simulink model "custom_springs_ALL"  (R2026a)
settings: Solver=ode23t  StopTime=15  AbsTol=1e-3  EnableMultiTasking=on
InitFcn:
  | warning off Simulink:SL_MatchingFromNotFound
  | m=1;
  | b=1;
  | k=1;
libraries: fl_lib x58, nesl_utility x10
Description:
  | Copyright 2014-2026 The MathWorks, Inc.
settings Model: Creator=tegel  LastModifiedBy=smiller
settings DataIOCC: SignalLoggingSaveFormat=ModelDataLogs
settings OptimizationCC: InitFltsAndDblsToZero=on
settings DebuggingCC: SaveWithParameterizedLinksMsg=none  UnderspecifiedInitializationDetection=Classic
settings HardwareCC: ProdHWDeviceType=32-bit Generic
settings GRTTargetCC: TargetFcnLib=ansi_tfl_tmw.mat  CombineOutputUpdateFcns=off  GRTInterface=on
settings SimscapeCC: SimscapeNormalizeSystem=off  SimscapeNominalValues="[{\"value\":\"1\",\"unit\":\"A\"},{\"value\":\"1\",\"unit\":\"bar\"},{\"value\":\"1\",\"unit\":\"cm^2\"},{\"value\":\"1\",\"unit\":\"cm^3/s\"},{\"value\":\"1\",\"unit\":\"kJ/kg\"},{\"value\":\"1\",\"unit\":\"kW\"},{\"value\":\"1\",\"unit\":\"l\"},{\"value\":\"1\",\"unit\":\"N\"},{\"value\":\"1\",\"unit\":\"N*m\"},{\"value\":\"1\",\"unit\":\"V\"}]"  SimscapeLogType=none  SimscapeLogDataHistory=5000.0

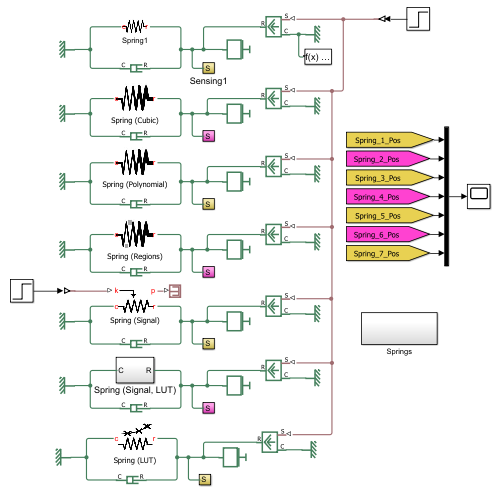
[thumbnail: Simulink's stored preview of the top-level diagram]
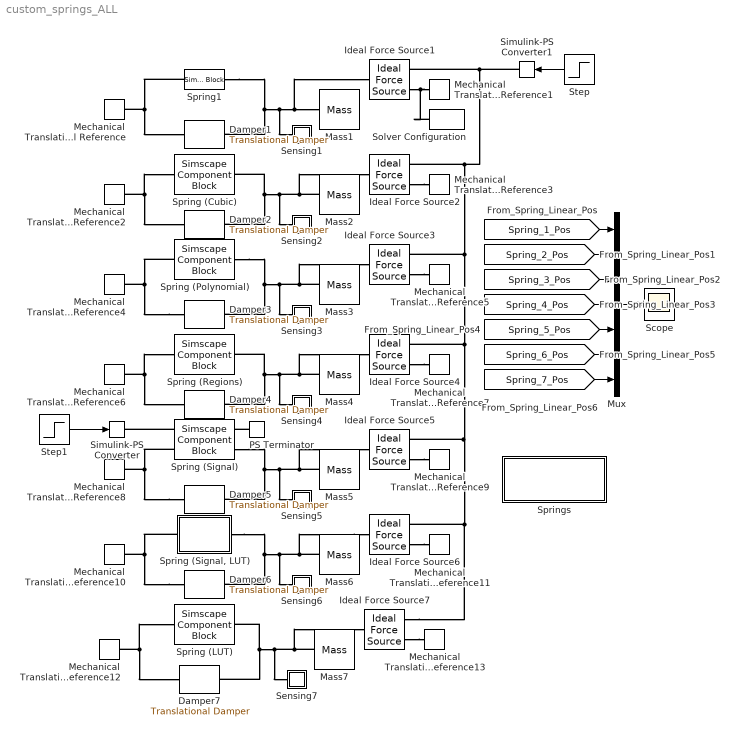
== system custom_springs_ALL ==
  Damper{1..7} (7 alike) : fl_lib/Mechanical/Translational Elements/Translational Damper  D=b N/(m/s)  v_specify=off  v_priority=High  v=0 m/s  v_nominal_specify=off  v_nominal_value=1  v_nominal_unit=m/s  f_specify=off  f_priority=High  f=0 N  f_nominal_specify=off  f_nominal_value=1  f_nominal_unit=N
  Ideal Force Source{1..7} (7 alike) : fl_lib/Mechanical/Mechanical Sources/Ideal Force Source
  Mass{1..7} (7 alike) : fl_lib/Mechanical/Translational Elements/Mass  mass=m kg  num_ports=foundation.enum.numPorts2.one  v_specify=on  v_priority=High  v=0 m/s  v_nominal_specify=off  v_nominal_value=1  v_nominal_unit=m/s  f_specify=off  f_priority=High  f=0 N  f_nominal_specify=off  f_nominal_value=1  f_nominal_unit=N
  Mechanical Translational Reference{,1..13} (14 alike) : fl_lib/Mechanical/Translational Elements/Mechanical Translational Reference
  Mux : Mux  Inputs=7
  PS Terminator : fl_lib/Physical Signals/Sinks/PS Terminator
  Scope : Scope
      settings: TimeSpan=15  ActiveDisplayYMinimum=0  ActiveDisplayYMaximum=2.5  DataLoggingVariableName=Simscape_Language_Spring_DATA
  Sensing1 : Subsystem
  Sensing2 : Subsystem
  Sensing3 : Subsystem
  Sensing4 : Subsystem
  Sensing5 : Subsystem
  Sensing6 : Subsystem
  Sensing7 : Subsystem
  Simulink-PS Converter : nesl_utility/Simulink-PS Converter  PhysicalDomain=network_engine_domain  SubClassName=ps_input  LeftPortType=input  RightPortType=output  PseudoPeriodic=off  Frequencies=[]  NoiseDistribution=none  NoiseParameters=[]  Unit=1  AffineConversion=off  FilteringAndDerivatives=provide  SimscapeFilterOrder=1  InputFilterTimeConstant=.001  UdotUserProvided=0
  Simulink-PS Converter1 : nesl_utility/Simulink-PS Converter  PhysicalDomain=network_engine_domain  SubClassName=ps_input  LeftPortType=input  RightPortType=output  PseudoPeriodic=off  Frequencies=[]  NoiseDistribution=none  NoiseParameters=[]  Unit=1  AffineConversion=off  FilteringAndDerivatives=provide  SimscapeFilterOrder=1  InputFilterTimeConstant=.001  UdotUserProvided=0
  Solver Configuration : nesl_utility/Solver Configuration  PhysicalDomain=network_engine_domain  SubClassName=solver  LeftPortType=input  RightPortType=generic  Tones=[]  Harmonics=[]  SimulateNoise=off  Profile=off  UseLocalSampling=off  EnableSwitchedLinearOptims=on  FrequencyDomain=off  UseCCode=off  RelTol=0.001  AbsTol=1e-06  MinStep=1e-09  ToWorkspace=off  RevertToSquareIcSolve=off  NumHomotopyIterations=100  PhasorMode=off  PhasorModeNumHarmonics=1  ConsistencySolver=NEWTON_FTOL  CanonicalOrdering=UNORDERED  OptimizeIntermediates=UNOPTIMIZED  IndexReductionMethod=DerivativeReplacement  DoDC=off  ResidualTolerance=1e-9  ConsistencyTolSource=GLOBAL  ConsistencyAbsTol=0.001  ConsistencyRelTol=0.001  ConsistencyTolFactor=0.001  UseLocalSolver=off  LocalSolverChoice=NE_BACKWARD_EULER_ADVANCER  ResolveIndetEquations=on  FunctionEvalNumThread=1  LocalSolverSampleTime=.001  DoFixedCost=off  MaxNonlinIter=3  MaxModeIter=2  ComputeImpulses=off  ImpulseIterations=2  LinearAlgebra=Sparse  LinearAlgebraNumThread=0  EquationFormulation=NE_TIME_EF  DelaysMemoryBudget=1024  AutomaticFiltering=on  FilteringTimeConstant=0.001  PartitionStorageMethod=AS_NEEDED  PartitionMemoryBudget=1024  PartitionMethod=FAST  MultibodyUseLocalSolver=off  MultibodyLocalSolverChoice=ODE1  MultibodyLocalSolverSampleTime=0.001
  Spring (Cubic) : SimscapeComponentBlock  SourceFile=CustomSprings.SpringCubic  ComponentPath=CustomSprings.SpringCubic  ComponentVariants=CustomSprings.SpringCubic  ComponentVariantNames=SpringCubic  ClassName=SpringCubic  SchemaVersion=1  k=1 N/m^3  v_specify=off  v_priority=None  v=0 m/s  v_nominal_specify=off  v_nominal_value=1  v_nominal_unit=m/s  f_specify=off  f_priority=None  f=0 N  f_nominal_specify=off  f_nominal_value=1  f_nominal_unit=N  x_specify=off  x_priority=None  x=0 m  x_nominal_specify=off  x_nominal_value=1  x_nominal_unit=m
      settings: CopyFcn=simscape.sscblock.internal.componentBlockCallback(gcbh,'COPY')  PreCopyFcn=simscape.sscblock.internal.componentBlockCallback(gcbh,'PRECOPY')  PreDeleteFcn=simscape.sscblock.internal.componentBlockCallback(gcbh,'PREDELETE')
      mask Type: Spring (Cubic)
  Spring (LUT) : SimscapeComponentBlock  SourceFile=CustomSprings.SpringLUT  ComponentPath=CustomSprings.SpringLUT  ComponentVariants=CustomSprings.SpringLUT  ComponentVariantNames=SpringLUT  ClassName=SpringLUT  SchemaVersion=1  xd=[-4.0, -3.0, -2.0, -1.0, 0.0, 1.0, 2.0, 3.0, 4.0] m  kd=[1000000.0, 8.0, 4.0, 2.0, 0.0, 2.0, 4.0, 8.0, 1000000.0] N/m  v_specify=off  v_priority=None  v=0 m/s  v_nominal_specify=off  v_nominal_value=1  v_nominal_unit=m/s  f_specify=off  f_priority=None  f=0 N  f_nominal_specify=off  f_nominal_value=1  f_nominal_unit=N  x_specify=off  x_priority=None  x=0 m  x_nominal_specify=off  x_nominal_value=1  x_nominal_unit=m  k_specify=off  k_priority=None  k=0 N/m  k_nominal_specify=off  k_nominal_value=1  k_nominal_unit=N/m
      settings: CopyFcn=simscape.sscblock.internal.componentBlockCallback(gcbh,'COPY')  PreCopyFcn=simscape.sscblock.internal.componentBlockCallback(gcbh,'PRECOPY')  PreDeleteFcn=simscape.sscblock.internal.componentBlockCallback(gcbh,'PREDELETE')
      mask Type: Spring (Lookup Table)
  Spring (Polynomial) : SimscapeComponentBlock  SourceFile=CustomSprings.SpringPolynomial  ComponentPath=CustomSprings.SpringPolynomial  ComponentVariants=CustomSprings.SpringPolynomial  ComponentVariantNames=SpringPolynomial  ClassName=SpringPolynomial  SchemaVersion=1  k=1 N/m  k1=1 N/m^3  v_specify=off  v_priority=None  v=0 m/s  v_nominal_specify=off  v_nominal_value=1  v_nominal_unit=m/s  f_specify=off  f_priority=None  f=0 N  f_nominal_specify=off  f_nominal_value=1  f_nominal_unit=N  x_specify=off  x_priority=None  x=0 m  x_nominal_specify=off  x_nominal_value=1  x_nominal_unit=m
      settings: CopyFcn=simscape.sscblock.internal.componentBlockCallback(gcbh,'COPY')  PreCopyFcn=simscape.sscblock.internal.componentBlockCallback(gcbh,'PRECOPY')  PreDeleteFcn=simscape.sscblock.internal.componentBlockCallback(gcbh,'PREDELETE')
      mask Type: Spring (Polynomial)
  Spring (Regions) : SimscapeComponentBlock  SourceFile=CustomSprings.SpringRegions  ComponentPath=CustomSprings.SpringRegions  ComponentVariants=CustomSprings.SpringRegions  ComponentVariantNames=SpringRegions  ClassName=SpringRegions  SchemaVersion=1  k=1 N/m  k1=1 N/m^3  xc=0.2 m  v_specify=off  v_priority=None  v=0 m/s  v_nominal_specify=off  v_nominal_value=1  v_nominal_unit=m/s  f_specify=off  f_priority=None  f=0 N  f_nominal_specify=off  f_nominal_value=1  f_nominal_unit=N  x_specify=off  x_priority=None  x=0 m  x_nominal_specify=off  x_nominal_value=1  x_nominal_unit=m
      settings: CopyFcn=simscape.sscblock.internal.componentBlockCallback(gcbh,'COPY')  PreCopyFcn=simscape.sscblock.internal.componentBlockCallback(gcbh,'PRECOPY')  PreDeleteFcn=simscape.sscblock.internal.componentBlockCallback(gcbh,'PREDELETE')
      mask Type: Spring (Regions)
  Spring (Signal) : SimscapeComponentBlock  SourceFile=CustomSprings.SpringSignal  ComponentPath=CustomSprings.SpringSignal  ComponentVariants=CustomSprings.SpringSignal  ComponentVariantNames=SpringSignal  ClassName=SpringSignal  SchemaVersion=1  v_specify=off  v_priority=None  v=0 m/s  v_nominal_specify=off  v_nominal_value=1  v_nominal_unit=m/s  f_specify=off  f_priority=None  f=0 N  f_nominal_specify=off  f_nominal_value=1  f_nominal_unit=N  x_specify=off  x_priority=None  x=0 m  x_nominal_specify=off  x_nominal_value=1  x_nominal_unit=m
      settings: CopyFcn=simscape.sscblock.internal.componentBlockCallback(gcbh,'COPY')  PreCopyFcn=simscape.sscblock.internal.componentBlockCallback(gcbh,'PRECOPY')  PreDeleteFcn=simscape.sscblock.internal.componentBlockCallback(gcbh,'PREDELETE')
      mask Type: Spring (Signal)
  "Spring (Signal, LUT)" : Subsystem
  Spring1 : SimscapeComponentBlock  SourceFile=CustomSprings.SpringLinear  ComponentPath=CustomSprings.SpringLinear  ComponentVariants=CustomSprings.SpringLinear  ComponentVariantNames=SpringLinear  ClassName=SpringLinear  SchemaVersion=1  k=1 N/m  v_specify=off  v_priority=None  v=0 m/s  v_nominal_specify=off  v_nominal_value=1  v_nominal_unit=m/s  f_specify=off  f_priority=None  f=0 N  f_nominal_specify=off  f_nominal_value=1  f_nominal_unit=N  x_specify=off  x_priority=None  x=0 m  x_nominal_specify=off  x_nominal_value=1  x_nominal_unit=m
      settings: CopyFcn=simscape.sscblock.internal.componentBlockCallback(gcbh,'COPY')  PreCopyFcn=simscape.sscblock.internal.componentBlockCallback(gcbh,'PRECOPY')  PreDeleteFcn=simscape.sscblock.internal.componentBlockCallback(gcbh,'PREDELETE')
      mask Type: Spring
  Springs : Subsystem
  Step : Step  FinalValue=2  SampleTime=0
  Step1 : Step  Time=10  InitialValue=1  FinalValue=2  SampleTime=0
  wires:
  Mux/1 -> Scope/1
  [Spring_1_Pos] -> Mux/1
  [Spring_2_Pos] -> Mux/2
  Step/1 -> Simulink-PS Converter1/1
  Step1/1 -> Simulink-PS Converter/1
  [Spring_3_Pos] -> Mux/3
  [Spring_4_Pos] -> Mux/4
  [Spring_5_Pos] -> Mux/5
  [Spring_6_Pos] -> Mux/6
  [Spring_7_Pos] -> Mux/7
  connections:
  Ideal Force Source4/RConn1 -- Ideal Force Source3/RConn1 -- Ideal Force Source1/RConn1 -- Simulink-PS Converter1/RConn1 -- Ideal Force Source2/RConn1 -- Ideal Force Source5/RConn1 -- Ideal Force Source6/RConn1 -- Ideal Force Source7/RConn1
  Ideal Force Source1/RConn2 -- Solver Configuration/RConn1 -- Mechanical Translational Reference1/LConn1
  Mechanical Translational Reference/LConn1 -- Spring1/LConn1 -- Damper1/RConn1
  Damper1/LConn1 -- Spring1/RConn1 -- Sensing1/LConn1 -- Mass1/LConn1 -- Ideal Force Source1/LConn1
  Mechanical Translational Reference2/LConn1 -- Spring (Cubic)/LConn1 -- Damper2/RConn1
  Damper2/LConn1 -- Spring (Cubic)/RConn1 -- Sensing2/LConn1 -- Mass2/LConn1 -- Ideal Force Source2/LConn1
  Ideal Force Source2/RConn2 -- Mechanical Translational Reference3/LConn1
  Damper3/RConn1 -- Spring (Polynomial)/LConn1 -- Mechanical Translational Reference4/LConn1
  Spring (Polynomial)/RConn1 -- Damper3/LConn1 -- Ideal Force Source3/LConn1 -- Mass3/LConn1 -- Sensing3/LConn1
  Ideal Force Source3/RConn2 -- Mechanical Translational Reference5/LConn1
  Mechanical Translational Reference6/LConn1 -- Spring (Regions)/LConn1 -- Damper4/RConn1
  Damper4/LConn1 -- Spring (Regions)/RConn1 -- Sensing4/LConn1 -- Mass4/LConn1 -- Ideal Force Source4/LConn1
  Ideal Force Source4/RConn2 -- Mechanical Translational Reference7/LConn1
  Damper5/RConn1 -- Spring (Signal)/LConn2 -- Mechanical Translational Reference8/LConn1
  Spring (Signal)/RConn2 -- Damper5/LConn1 -- Ideal Force Source5/LConn1 -- Mass5/LConn1 -- Sensing5/LConn1
  Ideal Force Source5/RConn2 -- Mechanical Translational Reference9/LConn1
  Damper6/RConn1 -- "Spring (Signal, LUT)"/LConn1 -- Mechanical Translational Reference10/LConn1
  Ideal Force Source6/LConn1 -- "Spring (Signal, LUT)"/RConn1 -- Damper6/LConn1 -- Sensing6/LConn1 -- Mass6/LConn1
  Ideal Force Source6/RConn2 -- Mechanical Translational Reference11/LConn1
  Spring (Signal)/LConn1 -- Simulink-PS Converter/RConn1
  Mechanical Translational Reference12/LConn1 -- Spring (LUT)/LConn1 -- Damper7/RConn1
  Damper7/LConn1 -- Spring (LUT)/RConn1 -- Sensing7/LConn1 -- Mass7/LConn1 -- Ideal Force Source7/LConn1
  Ideal Force Source7/RConn2 -- Mechanical Translational Reference13/LConn1
  PS Terminator/LConn1 -- Spring (Signal)/RConn1

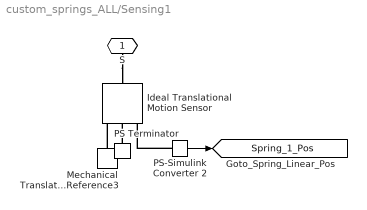
== system custom_springs_ALL/Sensing1 ==
  Ideal Translational Motion Sensor : fl_lib/Mechanical/Mechanical Sensors/Ideal Translational Motion Sensor  reference=foundation.enum.MeasurementReference.difference  acceleration_port=false  velocity_port=true  position_port=true  offset=0 m
  Mechanical Translational Reference3 : fl_lib/Mechanical/Translational Elements/Mechanical Translational Reference
  PS Terminator : fl_lib/Physical Signals/Sinks/PS Terminator
  PS-Simulink Converter 2 : nesl_utility/PS-Simulink Converter  PhysicalDomain=network_engine_domain  SubClassName=ps_output  LeftPortType=input  RightPortType=output  PseudoPeriodic=off  Frequencies=[]  VectorFormat=1-D array  Unit=1  AffineConversion=off
  S : PMIOPort  Side=Left
  tag scope: Spring_1_Pos=global
  wires:
  PS-Simulink Converter 2/1 -> [Spring_1_Pos]
  connections:
  S/RConn1 -- Ideal Translational Motion Sensor/LConn1
  Mechanical Translational Reference3/LConn1 -- Ideal Translational Motion Sensor/RConn1
  PS-Simulink Converter 2/LConn1 -- Ideal Translational Motion Sensor/RConn3
  PS Terminator/LConn1 -- Ideal Translational Motion Sensor/RConn2

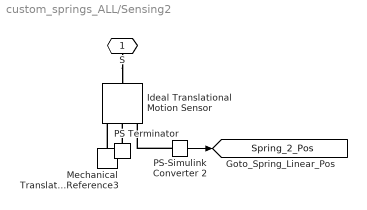
== system custom_springs_ALL/Sensing2 ==
  Ideal Translational Motion Sensor : fl_lib/Mechanical/Mechanical Sensors/Ideal Translational Motion Sensor  reference=foundation.enum.MeasurementReference.difference  acceleration_port=false  velocity_port=true  position_port=true  offset=0 m
  Mechanical Translational Reference3 : fl_lib/Mechanical/Translational Elements/Mechanical Translational Reference
  PS Terminator : fl_lib/Physical Signals/Sinks/PS Terminator
  PS-Simulink Converter 2 : nesl_utility/PS-Simulink Converter  PhysicalDomain=network_engine_domain  SubClassName=ps_output  LeftPortType=input  RightPortType=output  PseudoPeriodic=off  Frequencies=[]  VectorFormat=1-D array  Unit=1  AffineConversion=off
  S : PMIOPort  Side=Left
  tag scope: Spring_2_Pos=global
  wires:
  PS-Simulink Converter 2/1 -> [Spring_2_Pos]
  connections:
  PS-Simulink Converter 2/LConn1 -- Ideal Translational Motion Sensor/RConn3
  Mechanical Translational Reference3/LConn1 -- Ideal Translational Motion Sensor/RConn1
  S/RConn1 -- Ideal Translational Motion Sensor/LConn1
  PS Terminator/LConn1 -- Ideal Translational Motion Sensor/RConn2

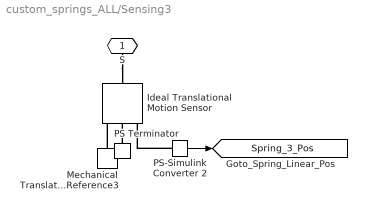
== system custom_springs_ALL/Sensing3 ==
  Ideal Translational Motion Sensor : fl_lib/Mechanical/Mechanical Sensors/Ideal Translational Motion Sensor  reference=foundation.enum.MeasurementReference.difference  acceleration_port=false  velocity_port=true  position_port=true  offset=0 m
  Mechanical Translational Reference3 : fl_lib/Mechanical/Translational Elements/Mechanical Translational Reference
  PS Terminator : fl_lib/Physical Signals/Sinks/PS Terminator
  PS-Simulink Converter 2 : nesl_utility/PS-Simulink Converter  PhysicalDomain=network_engine_domain  SubClassName=ps_output  LeftPortType=input  RightPortType=output  PseudoPeriodic=off  Frequencies=[]  VectorFormat=1-D array  Unit=1  AffineConversion=off
  S : PMIOPort  Side=Left
  tag scope: Spring_3_Pos=global
  wires:
  PS-Simulink Converter 2/1 -> [Spring_3_Pos]
  connections:
  S/RConn1 -- Ideal Translational Motion Sensor/LConn1
  Mechanical Translational Reference3/LConn1 -- Ideal Translational Motion Sensor/RConn1
  PS-Simulink Converter 2/LConn1 -- Ideal Translational Motion Sensor/RConn3
  PS Terminator/LConn1 -- Ideal Translational Motion Sensor/RConn2

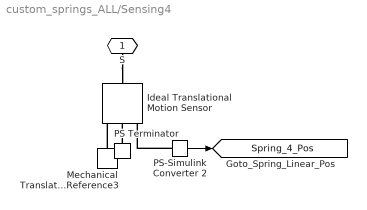
== system custom_springs_ALL/Sensing4 ==
  Ideal Translational Motion Sensor : fl_lib/Mechanical/Mechanical Sensors/Ideal Translational Motion Sensor  reference=foundation.enum.MeasurementReference.difference  acceleration_port=false  velocity_port=true  position_port=true  offset=0 m
  Mechanical Translational Reference3 : fl_lib/Mechanical/Translational Elements/Mechanical Translational Reference
  PS Terminator : fl_lib/Physical Signals/Sinks/PS Terminator
  PS-Simulink Converter 2 : nesl_utility/PS-Simulink Converter  PhysicalDomain=network_engine_domain  SubClassName=ps_output  LeftPortType=input  RightPortType=output  PseudoPeriodic=off  Frequencies=[]  VectorFormat=1-D array  Unit=1  AffineConversion=off
  S : PMIOPort  Side=Left
  tag scope: Spring_4_Pos=global
  wires:
  PS-Simulink Converter 2/1 -> [Spring_4_Pos]
  connections:
  PS-Simulink Converter 2/LConn1 -- Ideal Translational Motion Sensor/RConn3
  Mechanical Translational Reference3/LConn1 -- Ideal Translational Motion Sensor/RConn1
  S/RConn1 -- Ideal Translational Motion Sensor/LConn1
  PS Terminator/LConn1 -- Ideal Translational Motion Sensor/RConn2

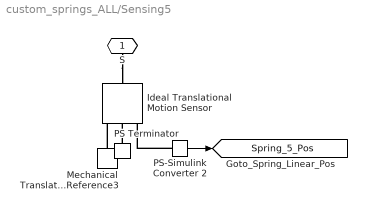
== system custom_springs_ALL/Sensing5 ==
  Ideal Translational Motion Sensor : fl_lib/Mechanical/Mechanical Sensors/Ideal Translational Motion Sensor  reference=foundation.enum.MeasurementReference.difference  acceleration_port=false  velocity_port=true  position_port=true  offset=0 m
  Mechanical Translational Reference3 : fl_lib/Mechanical/Translational Elements/Mechanical Translational Reference
  PS Terminator : fl_lib/Physical Signals/Sinks/PS Terminator
  PS-Simulink Converter 2 : nesl_utility/PS-Simulink Converter  PhysicalDomain=network_engine_domain  SubClassName=ps_output  LeftPortType=input  RightPortType=output  PseudoPeriodic=off  Frequencies=[]  VectorFormat=1-D array  Unit=1  AffineConversion=off
  S : PMIOPort  Side=Left
  tag scope: Spring_5_Pos=global
  wires:
  PS-Simulink Converter 2/1 -> [Spring_5_Pos]
  connections:
  S/RConn1 -- Ideal Translational Motion Sensor/LConn1
  Mechanical Translational Reference3/LConn1 -- Ideal Translational Motion Sensor/RConn1
  PS-Simulink Converter 2/LConn1 -- Ideal Translational Motion Sensor/RConn3
  PS Terminator/LConn1 -- Ideal Translational Motion Sensor/RConn2

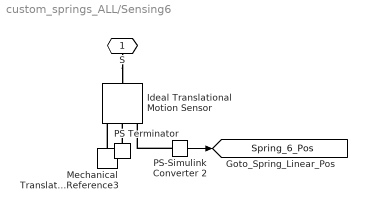
== system custom_springs_ALL/Sensing6 ==
  Ideal Translational Motion Sensor : fl_lib/Mechanical/Mechanical Sensors/Ideal Translational Motion Sensor  reference=foundation.enum.MeasurementReference.difference  acceleration_port=false  velocity_port=true  position_port=true  offset=0 m
  Mechanical Translational Reference3 : fl_lib/Mechanical/Translational Elements/Mechanical Translational Reference
  PS Terminator : fl_lib/Physical Signals/Sinks/PS Terminator
  PS-Simulink Converter 2 : nesl_utility/PS-Simulink Converter  PhysicalDomain=network_engine_domain  SubClassName=ps_output  LeftPortType=input  RightPortType=output  PseudoPeriodic=off  Frequencies=[]  VectorFormat=1-D array  Unit=1  AffineConversion=off
  S : PMIOPort  Side=Left
  tag scope: Spring_6_Pos=global
  wires:
  PS-Simulink Converter 2/1 -> [Spring_6_Pos]
  connections:
  PS-Simulink Converter 2/LConn1 -- Ideal Translational Motion Sensor/RConn3
  Mechanical Translational Reference3/LConn1 -- Ideal Translational Motion Sensor/RConn1
  S/RConn1 -- Ideal Translational Motion Sensor/LConn1
  PS Terminator/LConn1 -- Ideal Translational Motion Sensor/RConn2

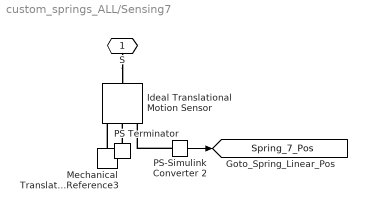
== system custom_springs_ALL/Sensing7 ==
  Ideal Translational Motion Sensor : fl_lib/Mechanical/Mechanical Sensors/Ideal Translational Motion Sensor  reference=foundation.enum.MeasurementReference.difference  acceleration_port=false  velocity_port=true  position_port=true  offset=0 m
  Mechanical Translational Reference3 : fl_lib/Mechanical/Translational Elements/Mechanical Translational Reference
  PS Terminator : fl_lib/Physical Signals/Sinks/PS Terminator
  PS-Simulink Converter 2 : nesl_utility/PS-Simulink Converter  PhysicalDomain=network_engine_domain  SubClassName=ps_output  LeftPortType=input  RightPortType=output  PseudoPeriodic=off  Frequencies=[]  VectorFormat=1-D array  Unit=1  AffineConversion=off
  S : PMIOPort  Side=Left
  tag scope: Spring_7_Pos=global
  wires:
  PS-Simulink Converter 2/1 -> [Spring_7_Pos]
  connections:
  S/RConn1 -- Ideal Translational Motion Sensor/LConn1
  Mechanical Translational Reference3/LConn1 -- Ideal Translational Motion Sensor/RConn1
  PS-Simulink Converter 2/LConn1 -- Ideal Translational Motion Sensor/RConn3
  PS Terminator/LConn1 -- Ideal Translational Motion Sensor/RConn2

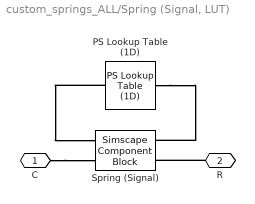
== system custom_springs_ALL/Spring (Signal, LUT) ==
  PS Lookup Table (1D) : fl_lib/Physical Signals/Lookup Tables/PS Lookup Table (1D)  x=[-4 -3 -2 -1 0 1 2 3 4] m  f=[1e6 8 4 2 0 2 4 8 1e6] N/m  interp_method=simscape.enum.interpolation.linear  extrap_method=simscape.enum.extrapolation.linear
  Spring (Signal) : SimscapeComponentBlock  SourceFile=CustomSprings.SpringSignal  ComponentPath=CustomSprings.SpringSignal  ComponentVariants=CustomSprings.SpringSignal  ComponentVariantNames=SpringSignal  ClassName=SpringSignal  SchemaVersion=1  v_specify=off  v_priority=None  v=0 m/s  v_nominal_specify=off  v_nominal_value=1  v_nominal_unit=m/s  f_specify=off  f_priority=None  f=0 N  f_nominal_specify=off  f_nominal_value=1  f_nominal_unit=N  x_specify=off  x_priority=None  x=0 m  x_nominal_specify=off  x_nominal_value=1  x_nominal_unit=m
      settings: CopyFcn=simscape.sscblock.internal.componentBlockCallback(gcbh,'COPY')  PreCopyFcn=simscape.sscblock.internal.componentBlockCallback(gcbh,'PRECOPY')  PreDeleteFcn=simscape.sscblock.internal.componentBlockCallback(gcbh,'PREDELETE')
      mask Type: Spring (Signal)
  C : PMIOPort  Side=Left
  R : PMIOPort  Port=2  Side=Right
  connections:
  PS Lookup Table (1D)/RConn1 -- Spring (Signal)/LConn1
  PS Lookup Table (1D)/LConn1 -- Spring (Signal)/RConn1
  C/RConn1 -- Spring (Signal)/LConn2
  R/RConn1 -- Spring (Signal)/RConn2

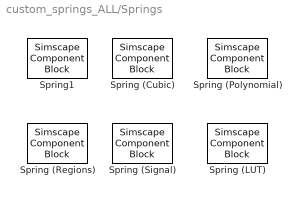
== system custom_springs_ALL/Springs ==
  Spring (Cubic) : SimscapeComponentBlock  SourceFile=CustomSprings.SpringCubic  ComponentPath=CustomSprings.SpringCubic  ComponentVariants=CustomSprings.SpringCubic  ComponentVariantNames=SpringCubic  ClassName=SpringCubic  SchemaVersion=1  k=1 N/m^3  v_specify=off  v_priority=None  v=0 m/s  v_nominal_specify=off  v_nominal_value=1  v_nominal_unit=m/s  f_specify=off  f_priority=None  f=0 N  f_nominal_specify=off  f_nominal_value=1  f_nominal_unit=N  x_specify=off  x_priority=None  x=0 m  x_nominal_specify=off  x_nominal_value=1  x_nominal_unit=m
      settings: CopyFcn=simscape.sscblock.internal.componentBlockCallback(gcbh,'COPY')  PreCopyFcn=simscape.sscblock.internal.componentBlockCallback(gcbh,'PRECOPY')  PreDeleteFcn=simscape.sscblock.internal.componentBlockCallback(gcbh,'PREDELETE')
      mask Type: Spring (Cubic)
  Spring (LUT) : SimscapeComponentBlock  SourceFile=CustomSprings.SpringLUT  ComponentPath=CustomSprings.SpringLUT  ComponentVariants=CustomSprings.SpringLUT  ComponentVariantNames=SpringLUT  ClassName=SpringLUT  SchemaVersion=1  xd=[-4.0, -3.0, -2.0, -1.0, 0.0, 1.0, 2.0, 3.0, 4.0] m  kd=[1000000.0, 8.0, 4.0, 2.0, 0.0, 2.0, 4.0, 8.0, 1000000.0] N/m  v_specify=off  v_priority=None  v=0 m/s  v_nominal_specify=off  v_nominal_value=1  v_nominal_unit=m/s  f_specify=off  f_priority=None  f=0 N  f_nominal_specify=off  f_nominal_value=1  f_nominal_unit=N  x_specify=off  x_priority=None  x=0 m  x_nominal_specify=off  x_nominal_value=1  x_nominal_unit=m  k_specify=off  k_priority=None  k=0 N/m  k_nominal_specify=off  k_nominal_value=1  k_nominal_unit=N/m
      settings: CopyFcn=simscape.sscblock.internal.componentBlockCallback(gcbh,'COPY')  PreCopyFcn=simscape.sscblock.internal.componentBlockCallback(gcbh,'PRECOPY')  PreDeleteFcn=simscape.sscblock.internal.componentBlockCallback(gcbh,'PREDELETE')
      mask Type: Spring (Lookup Table)
  Spring (Polynomial) : SimscapeComponentBlock  SourceFile=CustomSprings.SpringPolynomial  ComponentPath=CustomSprings.SpringPolynomial  ComponentVariants=CustomSprings.SpringPolynomial  ComponentVariantNames=SpringPolynomial  ClassName=SpringPolynomial  SchemaVersion=1  k=1 N/m  k1=1 N/m^3  v_specify=off  v_priority=None  v=0 m/s  v_nominal_specify=off  v_nominal_value=1  v_nominal_unit=m/s  f_specify=off  f_priority=None  f=0 N  f_nominal_specify=off  f_nominal_value=1  f_nominal_unit=N  x_specify=off  x_priority=None  x=0 m  x_nominal_specify=off  x_nominal_value=1  x_nominal_unit=m
      settings: CopyFcn=simscape.sscblock.internal.componentBlockCallback(gcbh,'COPY')  PreCopyFcn=simscape.sscblock.internal.componentBlockCallback(gcbh,'PRECOPY')  PreDeleteFcn=simscape.sscblock.internal.componentBlockCallback(gcbh,'PREDELETE')
      mask Type: Spring (Polynomial)
  Spring (Regions) : SimscapeComponentBlock  SourceFile=CustomSprings.SpringRegions  ComponentPath=CustomSprings.SpringRegions  ComponentVariants=CustomSprings.SpringRegions  ComponentVariantNames=SpringRegions  ClassName=SpringRegions  SchemaVersion=1  k=1 N/m  k1=1 N/m^3  xc=0.2 m  v_specify=off  v_priority=None  v=0 m/s  v_nominal_specify=off  v_nominal_value=1  v_nominal_unit=m/s  f_specify=off  f_priority=None  f=0 N  f_nominal_specify=off  f_nominal_value=1  f_nominal_unit=N  x_specify=off  x_priority=None  x=0 m  x_nominal_specify=off  x_nominal_value=1  x_nominal_unit=m
      settings: CopyFcn=simscape.sscblock.internal.componentBlockCallback(gcbh,'COPY')  PreCopyFcn=simscape.sscblock.internal.componentBlockCallback(gcbh,'PRECOPY')  PreDeleteFcn=simscape.sscblock.internal.componentBlockCallback(gcbh,'PREDELETE')
      mask Type: Spring (Regions)
  Spring (Signal) : SimscapeComponentBlock  SourceFile=CustomSprings.SpringSignal  ComponentPath=CustomSprings.SpringSignal  ComponentVariants=CustomSprings.SpringSignal  ComponentVariantNames=SpringSignal  ClassName=SpringSignal  SchemaVersion=1  v_specify=off  v_priority=None  v=0 m/s  v_nominal_specify=off  v_nominal_value=1  v_nominal_unit=m/s  f_specify=off  f_priority=None  f=0 N  f_nominal_specify=off  f_nominal_value=1  f_nominal_unit=N  x_specify=off  x_priority=None  x=0 m  x_nominal_specify=off  x_nominal_value=1  x_nominal_unit=m
      settings: CopyFcn=simscape.sscblock.internal.componentBlockCallback(gcbh,'COPY')  PreCopyFcn=simscape.sscblock.internal.componentBlockCallback(gcbh,'PRECOPY')  PreDeleteFcn=simscape.sscblock.internal.componentBlockCallback(gcbh,'PREDELETE')
      mask Type: Spring (Signal)
  Spring1 : SimscapeComponentBlock  SourceFile=CustomSprings.SpringLinear  ComponentPath=CustomSprings.SpringLinear  ComponentVariants=CustomSprings.SpringLinear  ComponentVariantNames=SpringLinear  ClassName=SpringLinear  SchemaVersion=1  k=1 N/m  v_specify=off  v_priority=None  v=0 m/s  v_nominal_specify=off  v_nominal_value=1  v_nominal_unit=m/s  f_specify=off  f_priority=None  f=0 N  f_nominal_specify=off  f_nominal_value=1  f_nominal_unit=N  x_specify=off  x_priority=None  x=0 m  x_nominal_specify=off  x_nominal_value=1  x_nominal_unit=m
      settings: CopyFcn=simscape.sscblock.internal.componentBlockCallback(gcbh,'COPY')  PreCopyFcn=simscape.sscblock.internal.componentBlockCallback(gcbh,'PRECOPY')  PreDeleteFcn=simscape.sscblock.internal.componentBlockCallback(gcbh,'PREDELETE')
      mask Type: Spring
